simulink model "Neurofeedback_Actual_getconnectivity"  (R2022a)
settings: Solver=VariableStepAuto  StartTime=0.0  StopTime=60  FixedStep=0.1  RelTol=1e-3
libraries: simulink x1
settings Model: SnapshotInterval=1  Creator=mariodelossantos  LastModifiedBy=mdls3
settings DebuggingCC: UnconnectedInputMsg=warning  UnconnectedOutputMsg=warning  UnconnectedLineMsg=warning
settings RTWCC: DLArmComputeVersion=19.05

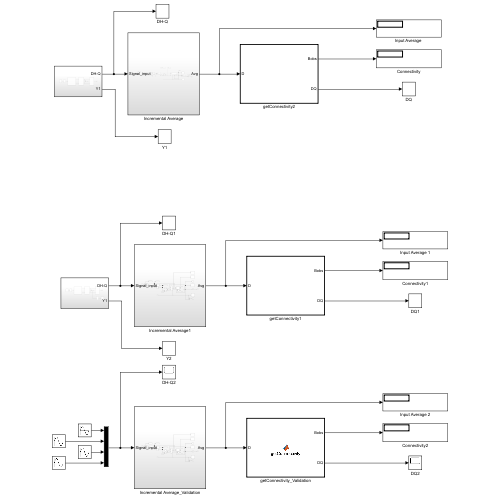
[thumbnail: Simulink's stored preview of the top-level diagram]
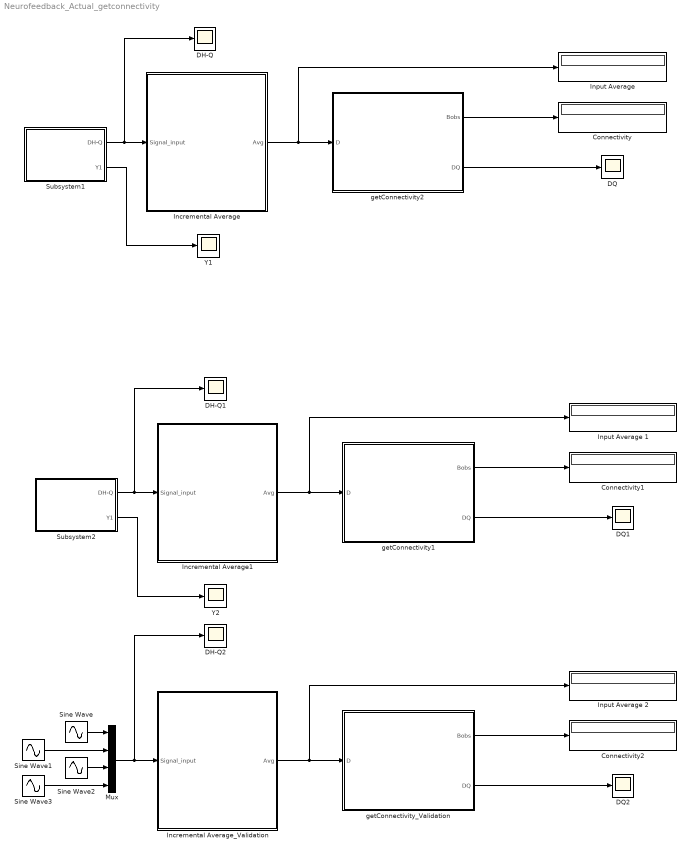
== system Neurofeedback_Actual_getconnectivity ==
  Connectivity : Display
  Connectivity1 : Display
  Connectivity2 : Display
  DH-Q : Scope
  DH-Q1 : Scope
  DH-Q2 : Scope
  DQ : Scope
  DQ1 : Scope
  DQ2 : Scope
  Incremental Average : Subsystem
  Incremental Average1 : Subsystem
  Incremental Average_Validation : Subsystem
  "Input Average " : Display
  Input Average 1 : Display
  Input Average 2 : Display
  Mux : Mux
  Sine Wave : Sin  SampleTime=0
  Sine Wave1 : Sin  Frequency=1.6  SampleTime=0
  Sine Wave2 : Sin  Frequency=0.8  SampleTime=0
  Sine Wave3 : Sin  Frequency=1.4  SampleTime=0
  Subsystem1 : Subsystem
  Subsystem2 : Subsystem
  Y1 : Scope
  Y2 : Scope
  getConnectivity1 : MATLAB Function  TreatAsAtomicUnit=on  SystemSampleTime=0
  getConnectivity2 : MATLAB Function  TreatAsAtomicUnit=on  SystemSampleTime=0
  getConnectivity_Validation : MATLAB Function  TreatAsAtomicUnit=on  SystemSampleTime=0
  wires:
  getConnectivity2/1(Bobs) -> Connectivity/1
  Incremental Average/1(Avg) -> getConnectivity2/1("D "), "Input Average "/1
  Subsystem1/1(DH-Q) -> DH-Q/1, Incremental Average/1(Signal_input)
  Subsystem1/2(Y1) -> Y1/1
  getConnectivity2/2(DQ) -> DQ/1
  Subsystem2/2(Y1) -> Y2/1
  Incremental Average1/1(Avg) -> getConnectivity1/1("D "), Input Average 1/1
  getConnectivity1/2(DQ) -> DQ1/1
  Subsystem2/1(DH-Q) -> DH-Q1/1, Incremental Average1/1(Signal_input)
  getConnectivity1/1(Bobs) -> Connectivity1/1
  Incremental Average_Validation/1(Avg) -> getConnectivity_Validation/1("D "), Input Average 2/1
  getConnectivity_Validation/1(Bobs) -> Connectivity2/1
  getConnectivity_Validation/2(DQ) -> DQ2/1
  Sine Wave/1 -> Mux/1
  Sine Wave1/1 -> Mux/2
  Sine Wave2/1 -> Mux/3
  Sine Wave3/1 -> Mux/4
  Mux/1 -> Incremental Average_Validation/1(Signal_input), DH-Q2/1

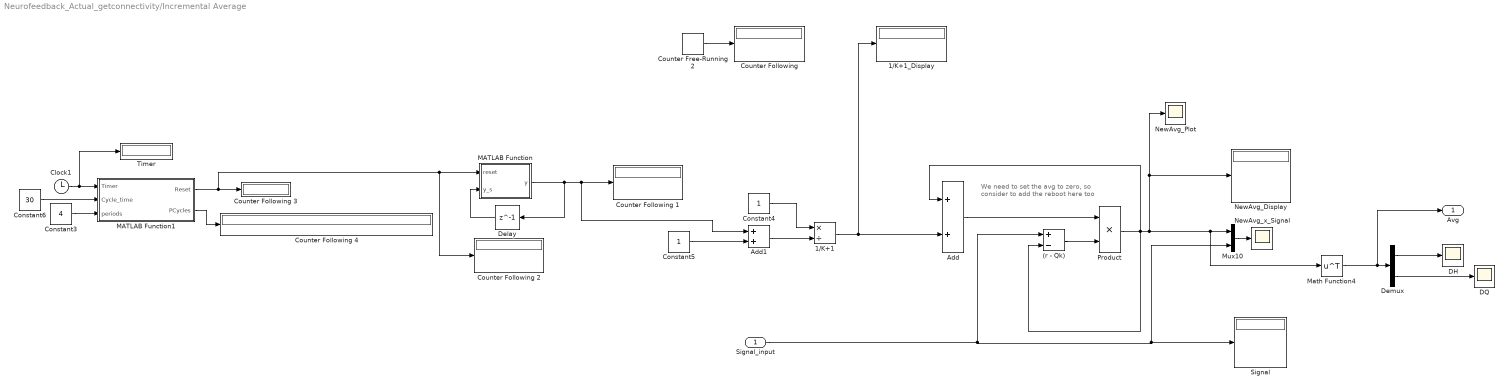
== system Neurofeedback_Actual_getconnectivity/Incremental Average ==
  note: We need to set the avg to zero, so consider to add the reboot here too
  Signal_input : Inport
  (r - Qk) : Sum  Inputs=+-
  1/K+1 : Product  Inputs=*/
  1/K+1_Display : Display
  Add : Sum
  Add1 : Sum
  Clock1 : Clock
  Constant3 : Constant  Value=4
  Constant4 : Constant
  Constant5 : Constant
  Constant6 : Constant  Value=30
  Counter Free-Running2 : simulink/Sources/Counter Free-Running  NumBits=16  tsamp=-1
  Counter Following {,1..4} (5 alike) : Display
  DH : Scope
  DQ : Scope
  Delay : Delay  DelayLength=1  InitialCondition=0
  Demux : Demux  Outputs=2
  MATLAB Function : MATLAB Function  TreatAsAtomicUnit=on
  MATLAB Function1 : MATLAB Function  TreatAsAtomicUnit=on
  Math Function4 : Math  Operator=transpose
  Mux10 : Mux  Inputs=2
  NewAvg_Display : Display
  NewAvg_Plot : Scope
  NewAvg_x_Signal : Scope
  Product : Product
  Signal : Display
  Timer : Display
  Avg : Outport
  wires:
  (r - Qk)/1 -> Product/2
  Signal_input/1 -> Signal/1, Mux10/2, (r - Qk)/1
  Add/1 -> Product/1
  Mux10/1 -> NewAvg_x_Signal/1
  Product/1 -> Add/1, (r - Qk)/2, NewAvg_Plot/1, NewAvg_Display/1, Math Function4/1, Mux10/1
  Math Function4/1 -> Avg/1, Demux/1
  Demux/2 -> DQ/1
  Demux/1 -> DH/1
  Constant4/1 -> 1/K+1/1
  Counter Free-Running2/1 -> "Counter Following "/1
  Constant5/1 -> Add1/2
  Add1/1 -> 1/K+1/2
  1/K+1/1 -> 1/K+1_Display/1, Add/2
  MATLAB Function/1(y) -> Add1/1, Counter Following 1/1, Delay/1
  Delay/1 -> MATLAB Function/2(y_s)
  MATLAB Function1/1(Reset) -> Counter Following 2/1, MATLAB Function/1(reset), Counter Following 3/1
  MATLAB Function1/2(PCycles) -> Counter Following 4/1
  Constant6/1 -> MATLAB Function1/2(Cycle_time)
  Constant3/1 -> MATLAB Function1/3(periods)
  Clock1/1 -> MATLAB Function1/1(Timer), Timer/1

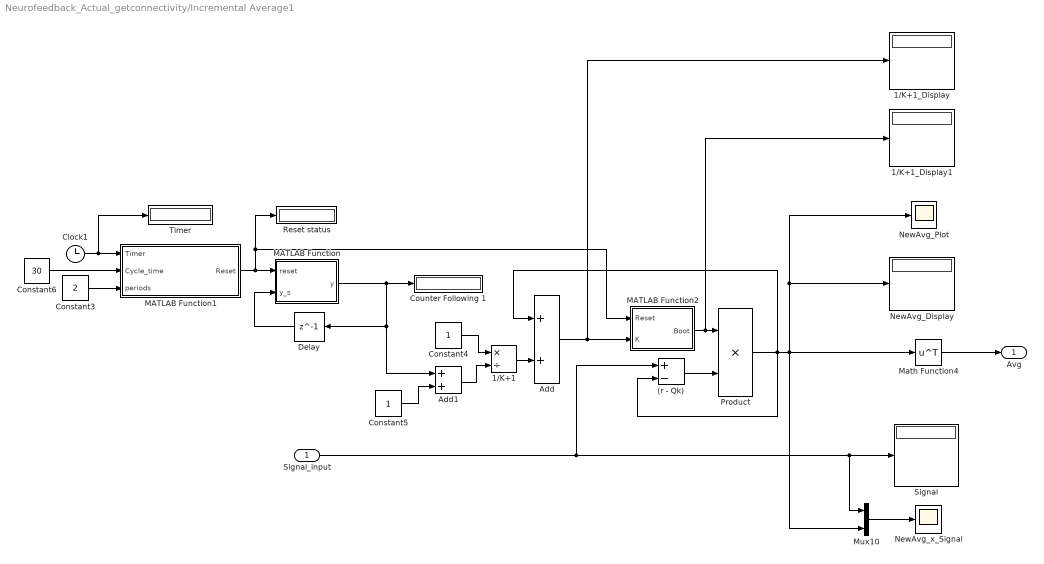
== system Neurofeedback_Actual_getconnectivity/Incremental Average1 ==
  Signal_input : Inport
  (r - Qk) : Sum  Inputs=+-
  1/K+1 : Product  Inputs=*/
  1/K+1_Display : Display
  1/K+1_Display1 : Display
  Add : Sum
  Add1 : Sum
  Clock1 : Clock
  Constant3 : Constant  Value=2
  Constant4 : Constant
  Constant5 : Constant
  Constant6 : Constant  Value=30
  Counter Following 1 : Display
  Delay : Delay  DelayLength=1  InitialCondition=0
  MATLAB Function : MATLAB Function  TreatAsAtomicUnit=on
  MATLAB Function1 : MATLAB Function  TreatAsAtomicUnit=on
  MATLAB Function2 : MATLAB Function  TreatAsAtomicUnit=on
  Math Function4 : Math  Operator=transpose
  Mux10 : Mux  Inputs=2
  NewAvg_Display : Display
  NewAvg_Plot : Scope
  NewAvg_x_Signal : Scope
  Product : Product
  Reset status : Display
  Signal : Display
  Timer : Display
  Avg : Outport
  wires:
  (r - Qk)/1 -> Product/2
  Signal_input/1 -> Mux10/1, Signal/1, (r - Qk)/1
  Add/1 -> 1/K+1_Display/1, MATLAB Function2/2(K)
  Mux10/1 -> NewAvg_x_Signal/1
  Product/1 -> Add/1, (r - Qk)/2, Mux10/2, NewAvg_Plot/1, NewAvg_Display/1, Math Function4/1
  Math Function4/1 -> Avg/1
  Constant4/1 -> 1/K+1/1
  Constant5/1 -> Add1/2
  Add1/1 -> 1/K+1/2
  1/K+1/1 -> Add/2
  MATLAB Function/1(y) -> Delay/1, Add1/1, Counter Following 1/1
  Delay/1 -> MATLAB Function/2(y_s)
  MATLAB Function1/1(Reset) -> Reset status/1, MATLAB Function2/1(Reset), MATLAB Function/1(reset)
  Constant6/1 -> MATLAB Function1/2(Cycle_time)
  Constant3/1 -> MATLAB Function1/3(periods)
  Clock1/1 -> MATLAB Function1/1(Timer), Timer/1
  MATLAB Function2/1(Boot) -> 1/K+1_Display1/1, Product/1

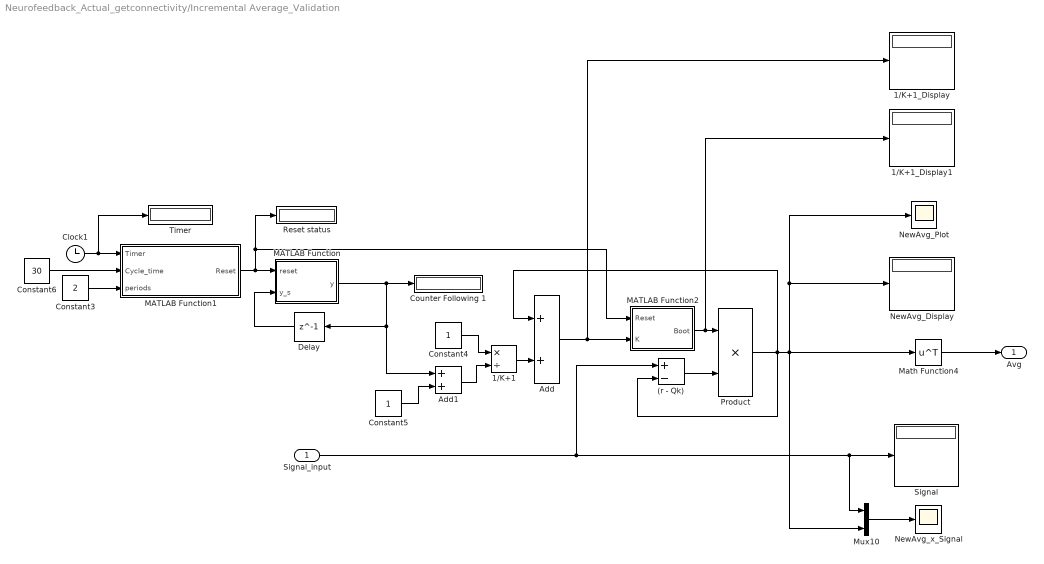
== system Neurofeedback_Actual_getconnectivity/Incremental Average_Validation ==
  Signal_input : Inport
  (r - Qk) : Sum  Inputs=+-
  1/K+1 : Product  Inputs=*/
  1/K+1_Display : Display
  1/K+1_Display1 : Display
  Add : Sum
  Add1 : Sum
  Clock1 : Clock
  Constant3 : Constant  Value=2
  Constant4 : Constant
  Constant5 : Constant
  Constant6 : Constant  Value=30
  Counter Following 1 : Display
  Delay : Delay  DelayLength=1  InitialCondition=0
  MATLAB Function : MATLAB Function  TreatAsAtomicUnit=on
  MATLAB Function1 : MATLAB Function  TreatAsAtomicUnit=on
  MATLAB Function2 : MATLAB Function  TreatAsAtomicUnit=on
  Math Function4 : Math  Operator=transpose
  Mux10 : Mux  Inputs=2
  NewAvg_Display : Display
  NewAvg_Plot : Scope
  NewAvg_x_Signal : Scope
  Product : Product
  Reset status : Display
  Signal : Display
  Timer : Display
  Avg : Outport
  wires:
  (r - Qk)/1 -> Product/2
  Signal_input/1 -> Mux10/1, Signal/1, (r - Qk)/1
  Add/1 -> 1/K+1_Display/1, MATLAB Function2/2(K)
  Mux10/1 -> NewAvg_x_Signal/1
  Product/1 -> Add/1, (r - Qk)/2, Mux10/2, NewAvg_Plot/1, NewAvg_Display/1, Math Function4/1
  Math Function4/1 -> Avg/1
  Constant4/1 -> 1/K+1/1
  Constant5/1 -> Add1/2
  Add1/1 -> 1/K+1/2
  1/K+1/1 -> Add/2
  MATLAB Function/1(y) -> Delay/1, Add1/1, Counter Following 1/1
  Delay/1 -> MATLAB Function/2(y_s)
  MATLAB Function1/1(Reset) -> Reset status/1, MATLAB Function2/1(Reset), MATLAB Function/1(reset)
  Constant6/1 -> MATLAB Function1/2(Cycle_time)
  Constant3/1 -> MATLAB Function1/3(periods)
  Clock1/1 -> MATLAB Function1/1(Timer), Timer/1
  MATLAB Function2/1(Boot) -> 1/K+1_Display1/1, Product/1

== system Neurofeedback_Actual_getconnectivity/Subsystem1 ==
  DH and DQ : Subsystem
  Hemodynamics : Subsystem
  Mux : Mux  Inputs=2
  Neurodynamics1 : Subsystem
  Optics : Subsystem
  Predefined_Stimulus : Subsystem
  DH-Q : Outport
  Y1 : Outport  Port=2
  wires:
  Mux/1 -> DH-Q/1
  Hemodynamics/1(Pj) -> DH and DQ/1(pj)
  Neurodynamics1/1(Z) -> Hemodynamics/1(Zj)  "Zj"
  Hemodynamics/2(qj) -> DH and DQ/2(qj)
  DH and DQ/1(DH) -> Mux/1, Optics/1(DH)
  Predefined_Stimulus/1(U) -> Neurodynamics1/1(U)
  Optics/1(Y1) -> Y1/1
  DH and DQ/2(DQ) -> Mux/2, Optics/2(DQ)

== system Neurofeedback_Actual_getconnectivity/Subsystem2 ==
  DH and DQ : Subsystem
  Display2 : Display
  Hemodynamics : Subsystem
  MATLAB Function : MATLAB Function  TreatAsAtomicUnit=on
  Mux : Mux  Inputs=2
  Neurodynamics1 : Subsystem
  Optics : Subsystem
  Predefined_Stimulus : Subsystem
  DH-Q : Outport
  Y1 : Outport  Port=2
  wires:
  Mux/1 -> MATLAB Function/1(DHQ), DH-Q/1
  Hemodynamics/1(Pj) -> DH and DQ/1(pj)
  Neurodynamics1/1(Z) -> Hemodynamics/1(Zj)  "Zj"
  Hemodynamics/2(qj) -> DH and DQ/2(qj)
  DH and DQ/1(DH) -> Mux/1, Optics/1(DH)
  Predefined_Stimulus/1(U) -> Neurodynamics1/1(U)
  Optics/1(Y1) -> Y1/1
  DH and DQ/2(DQ) -> Mux/2, Optics/2(DQ)
  MATLAB Function/1(Y) -> Display2/1

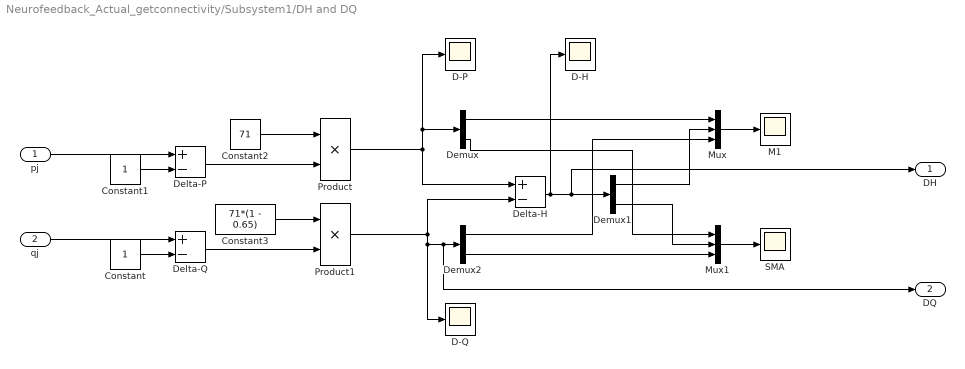
== system Neurofeedback_Actual_getconnectivity/Subsystem1/DH and DQ ==
  pj : Inport
  qj : Inport  Port=2
  Constant : Constant
  Constant1 : Constant
  Constant2 : Constant  Value=71
  Constant3 : Constant  Value=71*(1 - 0.65)
  D-H : Scope
  D-P : Scope
  D-Q : Scope
  Delta-H : Sum  Inputs=+-
  Delta-P : Sum  Inputs=+-
  Delta-Q : Sum  Inputs=+-
  Demux : Demux  Outputs=2
  Demux1 : Demux  Outputs=2
  Demux2 : Demux  Outputs=2
  M1 : Scope
  Mux : Mux  Inputs=3
  Mux1 : Mux  Inputs=3
  Product : Product
  Product1 : Product
  SMA : Scope
  DH : Outport
  DQ : Outport  Port=2
  wires:
  Constant2/1 -> Product/1
  Delta-Q/1 -> Product1/2
  Constant3/1 -> Product1/1
  Demux2/2 -> Mux1/3
  pj/1 -> Delta-P/1
  Mux1/1 -> SMA/1
  Demux/2 -> Mux1/1
  Mux/1 -> M1/1
  Constant/1 -> Delta-Q/2
  Delta-P/1 -> Product/2
  Product1/1 -> DQ/1, Demux2/1, D-Q/1, Delta-H/2
  qj/1 -> Delta-Q/1
  Demux/1 -> Mux/1
  Delta-H/1 -> DH/1, Demux1/1, D-H/1
  Demux1/1 -> Mux/2
  Demux1/2 -> Mux1/2
  Product/1 -> Demux/1, D-P/1, Delta-H/1
  Demux2/1 -> Mux/3
  Constant1/1 -> Delta-P/2

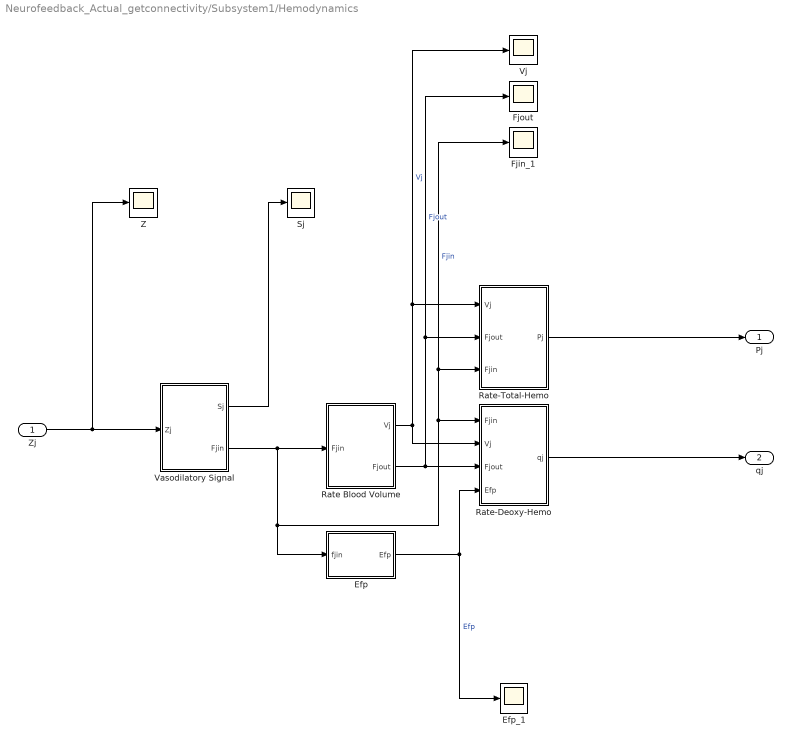
== system Neurofeedback_Actual_getconnectivity/Subsystem1/Hemodynamics ==
  Zj : Inport
  Efp : MATLAB Function  TreatAsAtomicUnit=on
  Efp_1 : Scope
  Fjin_1 : Scope
  Fjout : Scope
  Rate Blood Volume : Subsystem
  Rate-Deoxy-Hemo : Subsystem
  Rate-Total-Hemo : Subsystem
  Sj : Scope
  Vasodilatory Signal : Subsystem
  Vj : Scope
  Z : Scope
  Pj : Outport
  qj : Outport  Port=2
  wires:
  Rate-Deoxy-Hemo/1(qj) -> qj/1
  Zj/1 -> Vasodilatory Signal/1(Zj), Z/1
  Vasodilatory Signal/1(Sj) -> Sj/1
  Rate Blood Volume/2(Fjout) -> Fjout/1, Rate-Total-Hemo/2(Fjout), Rate-Deoxy-Hemo/3(Fjout)  "Fjout"
  Rate Blood Volume/1(Vj) -> Vj/1, Rate-Total-Hemo/1(Vj), Rate-Deoxy-Hemo/2(Vj)  "Vj"
  Rate-Total-Hemo/1(Pj) -> Pj/1
  Efp/1(Efp) -> Rate-Deoxy-Hemo/4(Efp), Efp_1/1  "Efp"
  Vasodilatory Signal/2(Fjin) -> Efp/1(fjin), Fjin_1/1, Rate-Total-Hemo/3(Fjin), Rate-Deoxy-Hemo/1(Fjin), Rate Blood Volume/1(Fjin)  "Fjin"

== system Neurofeedback_Actual_getconnectivity/Subsystem1/Neurodynamics1 ==
  U : Inport
  C : Gain  Gain=[0.08 0;0.06 0]  Multiplication=Matrix(K*u) (u vector)
  Integrator : Integrator
  Jt : MATLAB Function  TreatAsAtomicUnit=on
  MATLAB Function : MATLAB Function  TreatAsAtomicUnit=on
  MATLAB Function1 : MATLAB Function  TreatAsAtomicUnit=on
  Sum : Sum  Inputs=|++
  Z : Outport
  wires:
  Integrator/1 -> Z/1, Jt/1(Zt)
  C/1 -> Sum/1
  Jt/1(Jt) -> Sum/2
  U/1 -> Jt/2(U), MATLAB Function1/1(Z)
  Sum/1 -> MATLAB Function/1(Z)
  MATLAB Function/1(Zn) -> Integrator/1
  MATLAB Function1/1(Zn) -> C/1

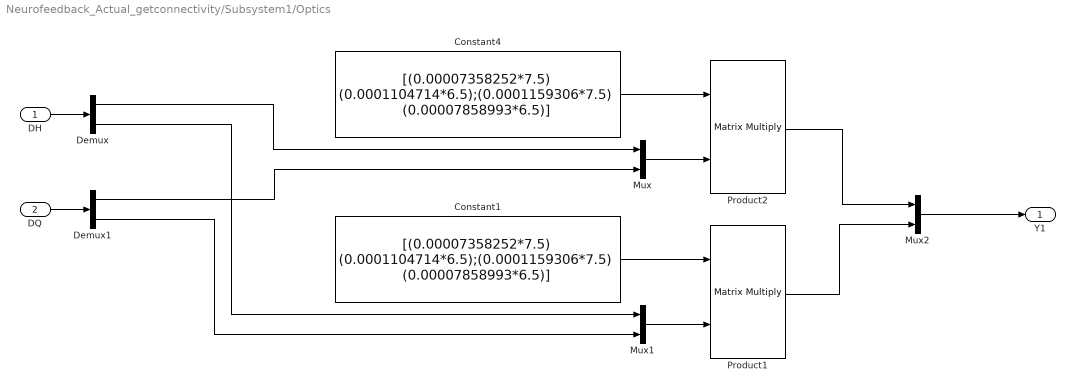
== system Neurofeedback_Actual_getconnectivity/Subsystem1/Optics ==
  DH : Inport
  DQ : Inport  Port=2
  Constant1 : Constant  Value=[(0.00007358252*7.5) (0.0001104714*6.5);(0.0001159306*7.5) (0.00007858993*6.5)]
  Constant4 : Constant  Value=[(0.00007358252*7.5) (0.0001104714*6.5);(0.0001159306*7.5) (0.00007858993*6.5)]
  Demux : Demux  Outputs=2
  Demux1 : Demux  Outputs=2
  Mux : Mux  Inputs=2
  Mux1 : Mux  Inputs=2
  Mux2 : Mux  Inputs=2
  Product1 : Product  Multiplication=Matrix(*)
  Product2 : Product  Multiplication=Matrix(*)
  Y1 : Outport
  wires:
  Mux/1 -> Product2/2
  Product2/1 -> Mux2/1
  Mux1/1 -> Product1/2
  Product1/1 -> Mux2/2
  Constant1/1 -> Product1/1
  DH/1 -> Demux/1
  Demux/1 -> Mux/1
  Demux/2 -> Mux1/1
  DQ/1 -> Demux1/1
  Constant4/1 -> Product2/1
  Demux1/1 -> Mux/2
  Demux1/2 -> Mux1/2
  Mux2/1 -> Y1/1

== system Neurofeedback_Actual_getconnectivity/Subsystem1/Predefined_Stimulus ==
  Mux : Mux  Inputs=2
  Pulse Generator : DiscretePulseGenerator  Amplitude=0.6  Period=30  PulseWidth=5
  Pulse Generator1 : DiscretePulseGenerator  Amplitude=0.6  Period=30  PulseWidth=6
  U : Outport
  wires:
  Mux/1 -> U/1
  Pulse Generator/1 -> Mux/1
  Pulse Generator1/1 -> Mux/2

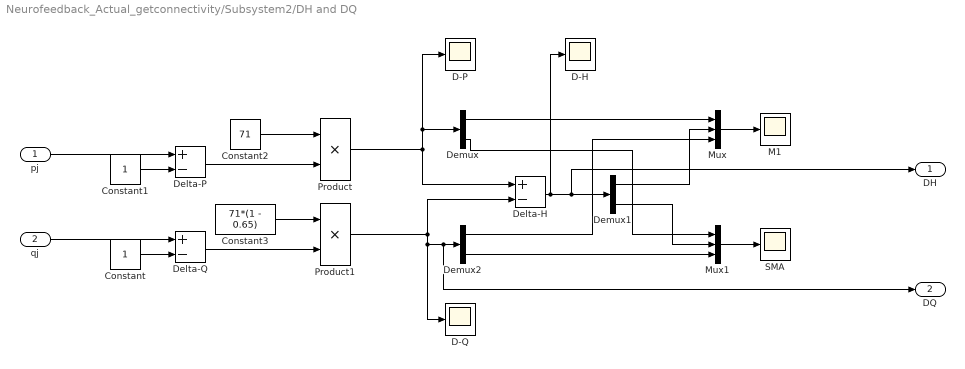
== system Neurofeedback_Actual_getconnectivity/Subsystem2/DH and DQ ==
  pj : Inport
  qj : Inport  Port=2
  Constant : Constant
  Constant1 : Constant
  Constant2 : Constant  Value=71
  Constant3 : Constant  Value=71*(1 - 0.65)
  D-H : Scope
  D-P : Scope
  D-Q : Scope
  Delta-H : Sum  Inputs=+-
  Delta-P : Sum  Inputs=+-
  Delta-Q : Sum  Inputs=+-
  Demux : Demux  Outputs=2
  Demux1 : Demux  Outputs=2
  Demux2 : Demux  Outputs=2
  M1 : Scope
  Mux : Mux  Inputs=3
  Mux1 : Mux  Inputs=3
  Product : Product
  Product1 : Product
  SMA : Scope
  DH : Outport
  DQ : Outport  Port=2
  wires:
  Constant2/1 -> Product/1
  Delta-Q/1 -> Product1/2
  Constant3/1 -> Product1/1
  Demux2/2 -> Mux1/3
  pj/1 -> Delta-P/1
  Mux1/1 -> SMA/1
  Demux/2 -> Mux1/1
  Mux/1 -> M1/1
  Constant/1 -> Delta-Q/2
  Delta-P/1 -> Product/2
  Product1/1 -> DQ/1, Demux2/1, D-Q/1, Delta-H/2
  qj/1 -> Delta-Q/1
  Demux/1 -> Mux/1
  Delta-H/1 -> DH/1, Demux1/1, D-H/1
  Demux1/1 -> Mux/2
  Demux1/2 -> Mux1/2
  Product/1 -> Demux/1, D-P/1, Delta-H/1
  Demux2/1 -> Mux/3
  Constant1/1 -> Delta-P/2

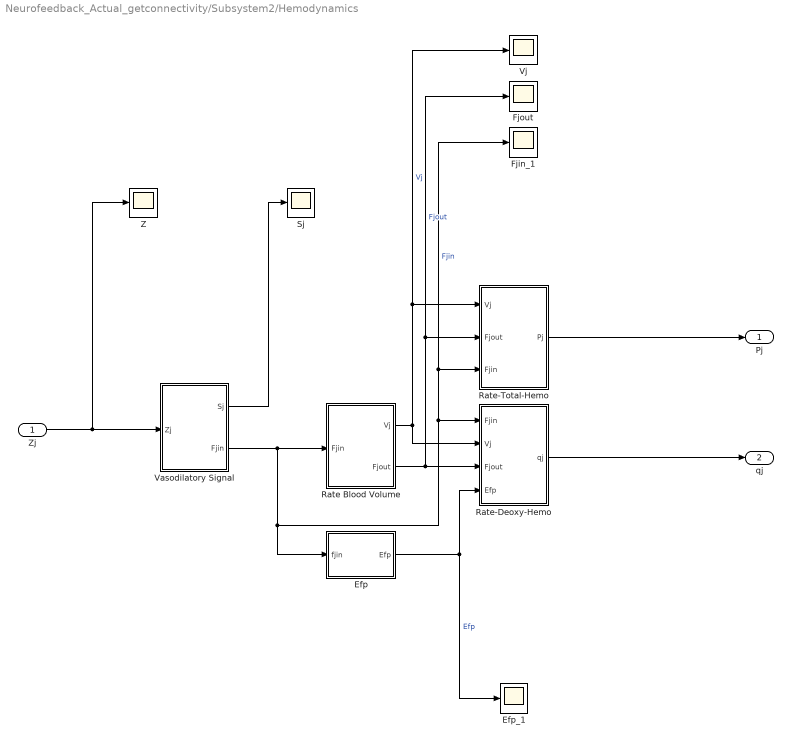
== system Neurofeedback_Actual_getconnectivity/Subsystem2/Hemodynamics ==
  Zj : Inport
  Efp : MATLAB Function  TreatAsAtomicUnit=on
  Efp_1 : Scope
  Fjin_1 : Scope
  Fjout : Scope
  Rate Blood Volume : Subsystem
  Rate-Deoxy-Hemo : Subsystem
  Rate-Total-Hemo : Subsystem
  Sj : Scope
  Vasodilatory Signal : Subsystem
  Vj : Scope
  Z : Scope
  Pj : Outport
  qj : Outport  Port=2
  wires:
  Rate-Deoxy-Hemo/1(qj) -> qj/1
  Zj/1 -> Vasodilatory Signal/1(Zj), Z/1
  Vasodilatory Signal/1(Sj) -> Sj/1
  Rate Blood Volume/2(Fjout) -> Fjout/1, Rate-Total-Hemo/2(Fjout), Rate-Deoxy-Hemo/3(Fjout)  "Fjout"
  Rate Blood Volume/1(Vj) -> Vj/1, Rate-Total-Hemo/1(Vj), Rate-Deoxy-Hemo/2(Vj)  "Vj"
  Rate-Total-Hemo/1(Pj) -> Pj/1
  Efp/1(Efp) -> Rate-Deoxy-Hemo/4(Efp), Efp_1/1  "Efp"
  Vasodilatory Signal/2(Fjin) -> Efp/1(fjin), Fjin_1/1, Rate-Total-Hemo/3(Fjin), Rate-Deoxy-Hemo/1(Fjin), Rate Blood Volume/1(Fjin)  "Fjin"

== system Neurofeedback_Actual_getconnectivity/Subsystem2/Neurodynamics1 ==
  U : Inport
  C : Gain  Gain=[0.08 0;0.06 0]  Multiplication=Matrix(K*u) (u vector)
  Integrator : Integrator
  Jt : MATLAB Function  TreatAsAtomicUnit=on
  MATLAB Function : MATLAB Function  TreatAsAtomicUnit=on
  MATLAB Function1 : MATLAB Function  TreatAsAtomicUnit=on
  Sum : Sum  Inputs=|++
  Z : Outport
  wires:
  Integrator/1 -> Z/1, Jt/1(Zt)
  C/1 -> Sum/1
  Jt/1(Jt) -> Sum/2
  U/1 -> Jt/2(U), MATLAB Function1/1(Z)
  Sum/1 -> MATLAB Function/1(Z)
  MATLAB Function/1(Zn) -> Integrator/1
  MATLAB Function1/1(Zn) -> C/1

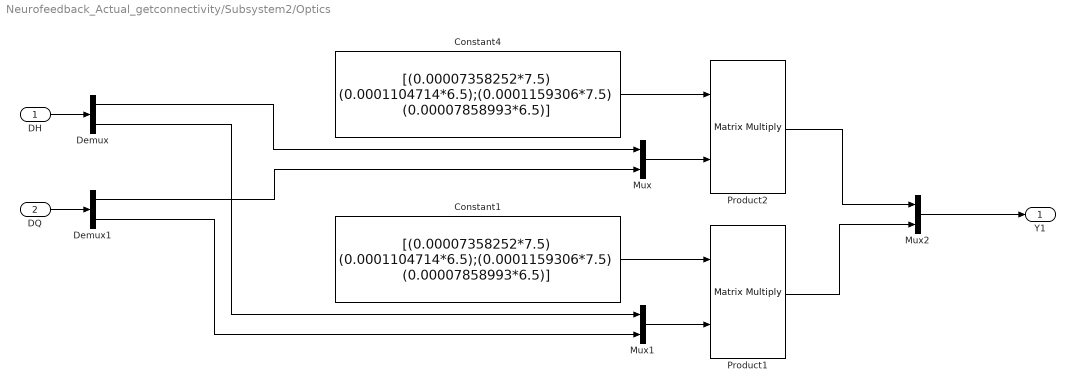
== system Neurofeedback_Actual_getconnectivity/Subsystem2/Optics ==
  DH : Inport
  DQ : Inport  Port=2
  Constant1 : Constant  Value=[(0.00007358252*7.5) (0.0001104714*6.5);(0.0001159306*7.5) (0.00007858993*6.5)]
  Constant4 : Constant  Value=[(0.00007358252*7.5) (0.0001104714*6.5);(0.0001159306*7.5) (0.00007858993*6.5)]
  Demux : Demux  Outputs=2
  Demux1 : Demux  Outputs=2
  Mux : Mux  Inputs=2
  Mux1 : Mux  Inputs=2
  Mux2 : Mux  Inputs=2
  Product1 : Product  Multiplication=Matrix(*)
  Product2 : Product  Multiplication=Matrix(*)
  Y1 : Outport
  wires:
  Mux/1 -> Product2/2
  Product2/1 -> Mux2/1
  Mux1/1 -> Product1/2
  Product1/1 -> Mux2/2
  Constant1/1 -> Product1/1
  DH/1 -> Demux/1
  Demux/1 -> Mux/1
  Demux/2 -> Mux1/1
  DQ/1 -> Demux1/1
  Constant4/1 -> Product2/1
  Demux1/1 -> Mux/2
  Demux1/2 -> Mux1/2
  Mux2/1 -> Y1/1

== system Neurofeedback_Actual_getconnectivity/Subsystem2/Predefined_Stimulus ==
  Mux : Mux  Inputs=2
  Pulse Generator : DiscretePulseGenerator  Amplitude=0.6  Period=30  PulseWidth=5
  Pulse Generator1 : DiscretePulseGenerator  Amplitude=0.6  Period=30  PulseWidth=6
  U : Outport
  wires:
  Mux/1 -> U/1
  Pulse Generator/1 -> Mux/1
  Pulse Generator1/1 -> Mux/2

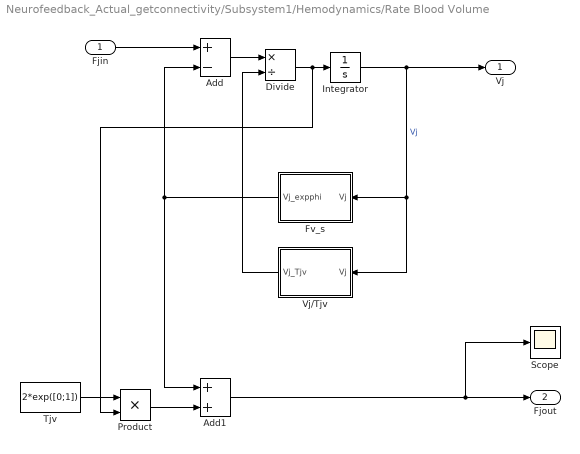
== system Neurofeedback_Actual_getconnectivity/Subsystem1/Hemodynamics/Rate Blood Volume ==
  Fjin : Inport
  Add : Sum  Inputs=+-
  Add1 : Sum
  Divide : Product  Inputs=*/
  Fv_s : MATLAB Function  TreatAsAtomicUnit=on
  Integrator : Integrator  InitialCondition=exp([0;0])
  Product : Product
  Scope : Scope
  Tjv : Constant  Value=2*exp([0;1])
  Vj/Tjv : MATLAB Function  TreatAsAtomicUnit=on
  Vj : Outport
  Fjout : Outport  Port=2
  wires:
  Fjin/1 -> Add/1
  Integrator/1 -> Vj/1, Vj/Tjv/1(Vj), Fv_s/1(Vj)  "Vj"
  Divide/1 -> Product/2, Integrator/1
  Fv_s/1(Vj_expphi) -> Add/2, Add1/1
  Add/1 -> Divide/1
  Vj/Tjv/1(Vj_Tjv) -> Divide/2
  Product/1 -> Add1/2
  Tjv/1 -> Product/1
  Add1/1 -> Scope/1, Fjout/1

== system Neurofeedback_Actual_getconnectivity/Subsystem1/Hemodynamics/Rate-Deoxy-Hemo ==
  Fjin : Inport
  Vj : Inport  Port=2
  Fjout : Inport  Port=3
  Efp : Inport  Port=4
  Divide : Product  Inputs=*/
  Integrator : Integrator  InitialCondition=exp([0;0])
  Product : Product
  Product1 : Product
  Subtract : Sum  Inputs=+-
  qj_scope : Scope
  qj : Outport
  wires:
  Efp/1 -> Product/2
  Divide/1 -> Product1/2
  Subtract/1 -> Integrator/1
  Integrator/1 -> qj/1, Divide/1, qj_scope/1
  Vj/1 -> Divide/2
  Product1/1 -> Subtract/2
  Fjin/1 -> Product/1
  Fjout/1 -> Product1/1
  Product/1 -> Subtract/1

== system Neurofeedback_Actual_getconnectivity/Subsystem1/Hemodynamics/Rate-Total-Hemo ==
  Vj : Inport
  Fjout : Inport  Port=2
  Fjin : Inport  Port=3
  Divide : Product  Inputs=*/
  Integrator : Integrator  InitialCondition=exp([0;0])
  Product : Product
  Subtract : Sum  Inputs=+-
  pj : Scope
  Pj : Outport
  wires:
  Fjout/1 -> Subtract/2
  Product/1 -> Integrator/1
  Vj/1 -> Divide/2
  Subtract/1 -> Product/1
  Fjin/1 -> Subtract/1
  Divide/1 -> Product/2
  Integrator/1 -> Pj/1, pj/1, Divide/1

== system Neurofeedback_Actual_getconnectivity/Subsystem1/Hemodynamics/Vasodilatory Signal ==
  Zj : Inport
  Add : Sum  Inputs=+--
  Add1 : Sum  Inputs=+-
  Constant1 : Constant
  Integrator : Integrator
  Integrator1 : Integrator  InitialCondition=exp([0;0])
  K : Gain  Gain=0.64*exp([0;0.05])
  Scope1 : Scope
  Yj : Gain  Gain=0.32*exp([0;0.05])
  Sj : Outport
  Fjin : Outport  Port=2
  wires:
  Add1/1 -> Yj/1
  K/1 -> Add/2  "Kj*Sj"
  Constant1/1 -> Add1/2
  Zj/1 -> Add/1
  Integrator1/1 -> Fjin/1, Scope1/1, Add1/1
  Integrator/1 -> Sj/1, K/1, Integrator1/1
  Add/1 -> Integrator/1
  Yj/1 -> Add/3  "Yj(Fjin - 1)"

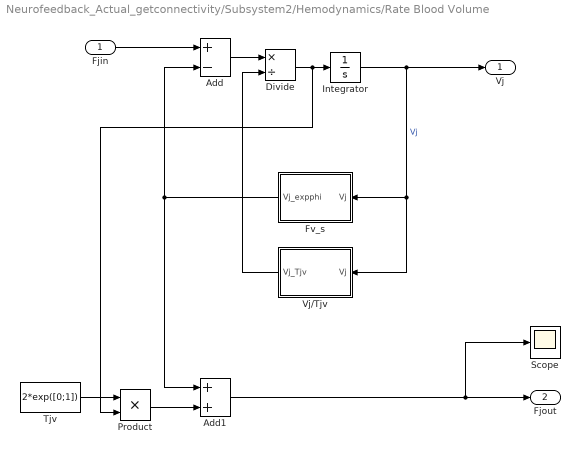
== system Neurofeedback_Actual_getconnectivity/Subsystem2/Hemodynamics/Rate Blood Volume ==
  Fjin : Inport
  Add : Sum  Inputs=+-
  Add1 : Sum
  Divide : Product  Inputs=*/
  Fv_s : MATLAB Function  TreatAsAtomicUnit=on
  Integrator : Integrator  InitialCondition=exp([0;0])
  Product : Product
  Scope : Scope
  Tjv : Constant  Value=2*exp([0;1])
  Vj/Tjv : MATLAB Function  TreatAsAtomicUnit=on
  Vj : Outport
  Fjout : Outport  Port=2
  wires:
  Fjin/1 -> Add/1
  Integrator/1 -> Vj/1, Vj/Tjv/1(Vj), Fv_s/1(Vj)  "Vj"
  Divide/1 -> Product/2, Integrator/1
  Fv_s/1(Vj_expphi) -> Add/2, Add1/1
  Add/1 -> Divide/1
  Vj/Tjv/1(Vj_Tjv) -> Divide/2
  Product/1 -> Add1/2
  Tjv/1 -> Product/1
  Add1/1 -> Scope/1, Fjout/1

== system Neurofeedback_Actual_getconnectivity/Subsystem2/Hemodynamics/Rate-Deoxy-Hemo ==
  Fjin : Inport
  Vj : Inport  Port=2
  Fjout : Inport  Port=3
  Efp : Inport  Port=4
  Divide : Product  Inputs=*/
  Integrator : Integrator  InitialCondition=exp([0;0])
  Product : Product
  Product1 : Product
  Subtract : Sum  Inputs=+-
  qj_scope : Scope
  qj : Outport
  wires:
  Efp/1 -> Product/2
  Divide/1 -> Product1/2
  Subtract/1 -> Integrator/1
  Integrator/1 -> qj/1, Divide/1, qj_scope/1
  Vj/1 -> Divide/2
  Product1/1 -> Subtract/2
  Fjin/1 -> Product/1
  Fjout/1 -> Product1/1
  Product/1 -> Subtract/1

== system Neurofeedback_Actual_getconnectivity/Subsystem2/Hemodynamics/Rate-Total-Hemo ==
  Vj : Inport
  Fjout : Inport  Port=2
  Fjin : Inport  Port=3
  Divide : Product  Inputs=*/
  Integrator : Integrator  InitialCondition=exp([0;0])
  Product : Product
  Subtract : Sum  Inputs=+-
  pj : Scope
  Pj : Outport
  wires:
  Fjout/1 -> Subtract/2
  Product/1 -> Integrator/1
  Vj/1 -> Divide/2
  Subtract/1 -> Product/1
  Fjin/1 -> Subtract/1
  Divide/1 -> Product/2
  Integrator/1 -> Pj/1, pj/1, Divide/1

== system Neurofeedback_Actual_getconnectivity/Subsystem2/Hemodynamics/Vasodilatory Signal ==
  Zj : Inport
  Add : Sum  Inputs=+--
  Add1 : Sum  Inputs=+-
  Constant1 : Constant
  Integrator : Integrator
  Integrator1 : Integrator  InitialCondition=exp([0;0])
  K : Gain  Gain=0.64*exp([0;0.05])
  Scope1 : Scope
  Yj : Gain  Gain=0.32*exp([0;0.05])
  Sj : Outport
  Fjin : Outport  Port=2
  wires:
  Add1/1 -> Yj/1
  K/1 -> Add/2  "Kj*Sj"
  Constant1/1 -> Add1/2
  Zj/1 -> Add/1
  Integrator1/1 -> Fjin/1, Scope1/1, Add1/1
  Integrator/1 -> Sj/1, K/1, Integrator1/1
  Add/1 -> Integrator/1
  Yj/1 -> Add/3  "Yj(Fjin - 1)"

== matlab function Neurofeedback_Actual_getconnectivity/Subsystem2/MATLAB Function ==
  data: DHQ input; Y output
function Y = Optics(DHQ)
%Adjust to the number of regions
Y = ones(1, 4);

F_P =[(0.0007358251*7.5) (0.001104715*6.5) ; (0.001159306*7.5) (0.0007858993*6.5)]; 

%Y(:,:) = F_P .*  DHQ;
 Y =  Y * 3;

== matlab function Neurofeedback_Actual_getconnectivity/Incremental Average_Validation/MATLAB Function ==
  data: reset input; y_s input; y output
function y = fcn(reset, y_s)

if reset == 1
    y = 0;
else 
    y = y_s + 1;
end

== matlab function Neurofeedback_Actual_getconnectivity/Incremental Average_Validation/MATLAB Function1 ==
  data: Timer input; Reset output; Cycle_time input; periods input
function Reset  = fcn(Timer, Cycle_time, periods)

temp = 0;
PCycles = zeros(periods,1);
for i = 1:periods
    PCycles(i) = i * Cycle_time;
    if (Timer >= PCycles(i) && Timer <= PCycles(i)+1)
        temp = 1;
        break
    else
        temp = 0;
    end
end 
Reset = temp;

== matlab function Neurofeedback_Actual_getconnectivity/Incremental Average/MATLAB Function ==
  data: reset input; y_s input; y output
function y = fcn(reset, y_s)

if reset == 1
    y = 0;
else 
    y = y_s + 1;
end

== matlab function Neurofeedback_Actual_getconnectivity/Incremental Average/MATLAB Function1 ==
  data: Timer input; Reset output; Cycle_time input; periods input; PCycles output
function [Reset, PCycles] = fcn(Timer, Cycle_time, periods)

temp = 0;
PCycles = zeros(4,1);
for i = 1:periods
    PCycles(i) = i * Cycle_time;
    if (Timer >= PCycles(i) && Timer <= PCycles(i)+1)
        temp = 1;
        break
    else
        temp = 0;
    end
end 
Reset = temp;

== matlab function Neurofeedback_Actual_getconnectivity/Incremental Average1/MATLAB Function ==
  data: reset input; y_s input; y output
function y = fcn(reset, y_s)

if reset == 1
    y = 0;
else 
    y = y_s + 1;
end

== matlab function Neurofeedback_Actual_getconnectivity/Subsystem1/Hemodynamics/Rate Blood Volume/Vj//Tjv ==
  data: Vj input; Vj_Tjv output
function Vj_Tjv = fcn(Vj)
    Tjv = 2*exp([0;1]);
    Tj = 2*exp([0;0.05]);
Vj_Tjv =(Tj.*Tjv.*Vj);

== matlab function Neurofeedback_Actual_getconnectivity/Subsystem1/Neurodynamics1/Jt ==
  data: Zt input; U input; Jt output
function Jt = fcn(Zt, U)
   A = [-0.16 -0.49;-0.02 -0.33];
   nRegions  = size(A,1);
   M = size(U,1); %nStimuli
   simulationLength = size(U,2);
   B = zeros(2,2,2);
   B1 = [0 0; 0 0]; %There must be a B per stimulus
   B2 = [-0.02 -0.77; 0.33 -1.31];
   B(:,:,1) = B1;
   B(:,:,2) = B2;
      assert(M == size(B,3),...
       'Unexpected number of induced connectivity parameters B.');
   T = zeros(nRegions); %nRegions x nRegions
    for t = 1:simulationLength
           for uu = 1:M % Sum (Uj * Bj)
               tmp = U(uu,t)*B(:,:,uu);
               T = -0.5*exp(T + tmp);  
           end
    end
    SI = diag(A);
    A =  A - diag(exp(SI) + (SI));
Jt = (A*Zt) + (T*Zt);

== matlab function Neurofeedback_Actual_getconnectivity/Subsystem1/Neurodynamics1/MATLAB Function ==
  data: Z input; Zn output
function Zn = fcn(Z)

Zn = Z(:,1);

== matlab function Neurofeedback_Actual_getconnectivity/Subsystem1/Neurodynamics1/MATLAB Function1 ==
  data: Z input; Zn output
function Zn = fcn(Z)

Zn = Z(:,1);

== matlab function Neurofeedback_Actual_getconnectivity/getConnectivity2 ==
  data: D input; Bobs output; DQ output
function [Bobs,DQ]  = getConnectivity(D)

    DQ = zeros(1, 2);
    DQ(1,1)=D(1,1);
    DQ(1,2)=D(1,2);


    DH = zeros(1,2);
    DH(1,1)=D(1,3);
    DH(1,2)=D(1,4);
    rThresh= 0.4; % [0..1] A threshold on the correlation.

    [nSamples, nChannels, nHb]=size(D);

    C = nan(nChannels, nChannels, nHb); %Matrix of channel pairwise correlations;


    %This part of the algorithm is HIGHLY inefficient but it does the job for now
    %but might not be sufficiently fast for "real time" neurofeedback

    for iHb = 1:nHb
        for iCh=1:nChannels
            for jCh=iCh:nChannels

                if iCh == jCh

                 C(iCh,jCh,iHb) = 1;

               else

                 C(iCh,jCh,iHb) = xcorr2(D(:,iCh,iHb),D(:,jCh,iHb));

                end
            end

        end

    end

    %Threshold/Binarize C


    tmp = C > rThresh;

    %Finally "merge" accross Hb species

    Bobs = all(tmp,3); %Apply the AND function across Hb species.

== matlab function Neurofeedback_Actual_getconnectivity/Incremental Average_Validation/MATLAB Function2 ==
  data: Reset input; K input; Boot output
function Boot = fcn(Reset, K)

    temp = ones(4, 1);
    Boot = [0;0;0;0];
    if Reset == 1
        temp = Boot;
    else 
        temp = K;
    end 

    Boot = temp;

== matlab function Neurofeedback_Actual_getconnectivity/getConnectivity_Validation ==
  data: D input; Bobs output; DQ output
function [Bobs,DQ]  = getConnectivity(D)

    DQ = zeros(1, 2);
    DQ(1,1)=D(1,1);
    DQ(1,2)=D(1,2);


    DH = zeros(1,2);
    DH(1,1)=D(1,3);
    DH(1,2)=D(1,4);

    rThresh= 0.6; % [0..1] A threshold on the correlation.

    [nSamples, nChannels, nHb]=size(DQ);

    C = nan(nChannels, nChannels, nHb); %Matrix of channel pairwise correlations;

    %This part of the algorithm is HIGHLY inefficient but it does the job for now
    %but might not be sufficiently fast for "real time" neurofeedback

    for iHb = 1:nHb
        for iCh=1:nChannels
            for jCh=iCh:nChannels

                if iCh == jCh

                 C(iCh,jCh,iHb) = 1;

               else

                 C(iCh,jCh,iHb) = xcorr2(DQ(:,iCh,iHb),DQ(:,jCh,iHb));

                end
            end

        end

    end

    %Threshold/Binarize C


    tmp = C > rThresh;

    %Finally "merge" accross Hb species

    Bobs = all(tmp,3); %Apply the AND function across Hb species.

== matlab function Neurofeedback_Actual_getconnectivity/Incremental Average1/MATLAB Function1 ==
  data: Timer input; Reset output; Cycle_time input; periods input
function Reset  = fcn(Timer, Cycle_time, periods)

temp = 0;
PCycles = zeros(periods,1);
for i = 1:periods
    PCycles(i) = i * Cycle_time;
    if (Timer >= PCycles(i) && Timer <= PCycles(i)+1)
        temp = 1;
        break
    else
        temp = 0;
    end
end 
Reset = temp;

== matlab function Neurofeedback_Actual_getconnectivity/Subsystem2/Hemodynamics/Efp ==
  data: fjin input; Efp output
function Efp= fcn(fjin)

Efp = (1 - (1 - 0.32).^ (1 ./ fjin))/0.32;

== matlab function Neurofeedback_Actual_getconnectivity/Subsystem2/Hemodynamics/Rate Blood Volume/Fv_s ==
  data: Vj input; Vj_expphi output
function Vj_expphi = fcn(Vj)
phi = 0.32;
Vj_expphi = Vj.^(1/phi);

== matlab function Neurofeedback_Actual_getconnectivity/Subsystem2/Hemodynamics/Rate Blood Volume/Vj//Tjv ==
  data: Vj input; Vj_Tjv output
function Vj_Tjv = fcn(Vj)
    Tjv = 2*exp([0;1]);
    Tj = 2*exp([0;0.05]);
Vj_Tjv =(Tj.*Tjv.*Vj);

== matlab function Neurofeedback_Actual_getconnectivity/Subsystem2/Neurodynamics1/Jt ==
  data: Zt input; U input; Jt output
function Jt = fcn(Zt, U)
   A = [-0.16 -0.49;-0.02 -0.33];
   nRegions  = size(A,1);
   M = size(U,1); %nStimuli
   simulationLength = size(U,2);
   B = zeros(2,2,2);
   B1 = [0 0; 0 0]; %There must be a B per stimulus
   B2 = [-0.02 -0.77; 0.33 -1.31];
   B(:,:,1) = B1;
   B(:,:,2) = B2;
      assert(M == size(B,3),...
       'Unexpected number of induced connectivity parameters B.');
   T = zeros(nRegions); %nRegions x nRegions
    for t = 1:simulationLength
           for uu = 1:M % Sum (Uj * Bj)
               tmp = U(uu,t)*B(:,:,uu);
               T = -0.5*exp(T + tmp);  
           end
    end
    SI = diag(A);
    A =  A - diag(exp(SI) + (SI));
Jt = (A*Zt) + (T*Zt);

== matlab function Neurofeedback_Actual_getconnectivity/Subsystem2/Neurodynamics1/MATLAB Function ==
  data: Z input; Zn output
function Zn = fcn(Z)

Zn = Z(:,1);

== matlab function Neurofeedback_Actual_getconnectivity/Subsystem2/Neurodynamics1/MATLAB Function1 ==
  data: Z input; Zn output
function Zn = fcn(Z)

Zn = Z(:,1);

== matlab function Neurofeedback_Actual_getconnectivity/getConnectivity1 ==
  data: D input; Bobs output; DQ output
function [Bobs,DQ]  = getConnectivity(D)

    DQ = zeros(1, 2);
    DQ(1,1)=D(1,1);
    DQ(1,2)=D(1,2);


    DH = zeros(1,2);
    DH(1,1)=D(1,3);
    DH(1,2)=D(1,4);

    rThresh= 0.6; % [0..1] A threshold on the correlation.

    [nSamples, nChannels, nHb]=size(DQ);

    C = nan(nChannels, nChannels, nHb); %Matrix of channel pairwise correlations;

    %This part of the algorithm is HIGHLY inefficient but it does the job for now
    %but might not be sufficiently fast for "real time" neurofeedback

    for iHb = 1:nHb
        for iCh=1:nChannels
            for jCh=iCh:nChannels

                if iCh == jCh

                 C(iCh,jCh,iHb) = 1;

               else

                 C(iCh,jCh,iHb) = xcorr2(DQ(:,iCh,iHb),DQ(:,jCh,iHb));

                end
            end

        end

    end

    %Threshold/Binarize C


    tmp = C > rThresh;

    %Finally "merge" accross Hb species

    Bobs = all(tmp,3); %Apply the AND function across Hb species.

== matlab function Neurofeedback_Actual_getconnectivity/Incremental Average1/MATLAB Function2 ==
  data: Reset input; K input; Boot output
function Boot = fcn(Reset, K)

    temp = ones(4, 1);
    Boot = [0;0;0;0];
    if Reset == 1
        temp = Boot;
    else 
        temp = K;
    end 

    Boot = temp;

== matlab function Neurofeedback_Actual_getconnectivity/Subsystem1/Hemodynamics/Efp ==
  data: fjin input; Efp output
function Efp= fcn(fjin)

Efp = (1 - (1 - 0.32).^ (1 ./ fjin))/0.32;

== matlab function Neurofeedback_Actual_getconnectivity/Subsystem1/Hemodynamics/Rate Blood Volume/Fv_s ==
  data: Vj input; Vj_expphi output
function Vj_expphi = fcn(Vj)
phi = 0.32;
Vj_expphi = Vj.^(1/phi);
